simulink library "CDH_command_lib"  (R2018b)
settings: Solver=VariableStepAuto  StartTime=0.0  StopTime=10.0  RelTol=1e-3
undefined symbols (not defined in the file): fswParams
libraries: clock_lib x1
settings Model: Creator=colem  LastModifiedBy=colem

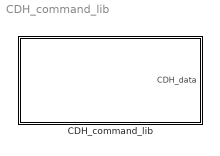
== system CDH_command_lib ==
  CDH_command_lib : Subsystem

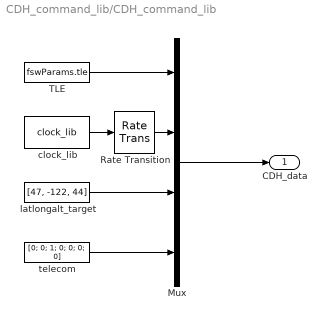
== system CDH_command_lib/CDH_command_lib ==
  Mux : Mux
  Rate Transition : RateTransition  OutPortSampleTime=fswParams.sample_time_s
  TLE : Constant  Value=fswParams.tle  SampleTime=fswParams.sample_time_s
  clock_lib : clock_lib/clock_lib  SystemSampleTime=-1
  latlongalt_target : Constant  Value=[47, -122, 44]  SampleTime=fswParams.sample_time_s
  telecom : Constant  Value=[0; 0; 1; 0; 0; 0; 0]  SampleTime=fswParams.sample_time_s
  CDH_data : Outport
  wires:
  clock_lib/1 -> Rate Transition/1
  TLE/1 -> Mux/1
  Mux/1 -> CDH_data/1
  latlongalt_target/1 -> Mux/3
  telecom/1 -> Mux/4
  Rate Transition/1 -> Mux/2
